simulink library "bcm"  (R2021b)
settings: Solver=VariableStepAuto  StartTime=0.0  StopTime=10.0  RelTol=1e-3
undefined symbols (not defined in the file or in its folder): ENUM_ANTITHEFT_ALARM, ENUM_ANTITHEFT_ARM, ENUM_ANTITHEFT_DISARM, ENUM_ANTITHEFT_WAIT, ENUM_GEARPOSNTOCAN_P, ENUM_PDKEYRAWLULOCK_INUNLOCK, ENUM_PDKEYRAWPS_INPS, ENUM_POWERSTA_ON, ENUM_POWERSTA_READY, ENUM_POWERSTA_STANDBY, ENUM_PWRSTASW_ON, ENUM_PWRSTASW_READY, ENUM_VEHICLETYPE_D21, ENUM_VEHICLETYPE_D31F25, ENUM_VEHICLETYPE_D31HAWD, ENUM_VEHICLETYPE_D31HRWD, ENUM_VEHICLETYPE_D31L24, FALSE, KBCM_ACCSwcPrsTmr_s, KBCM_ALMBrightnessDark_enum, KBCM_AmbBlue_enum, KBCM_AmbBreathT_ms, KBCM_AmbGreen_enum, KBCM_AmbMidPple_enum, KBCM_AmbRed_enum, KBCM_AmbTempCtrlEN_flg, KBCM_AmbTempT_s, KBCM_AmbWelModeENWait_s, KBCM_Antitheft_enum_ovrdflg, KBCM_Antitheft_enum_ovrdval, KBCM_APMDoorCtrlSta_flg_ovrdflg, KBCM_APMDoorCtrlSta_flg_ovrdval, KBCM_CmdKeepT_s, KBCM_CSWLightRstDebT_s, KBCM_CSWTurnLPRstT_s, KBCM_DelayTSW_flg, KBCM_DiagDRLOFF_flg, KBCM_DiagFLTC_mA, KBCM_DiagFMHT_s, KBCM_DiagFRTC_mA, KBCM_DiagRLTC_mA, KBCM_DiagRRTC_mA, KBCM_DrAPMRetryTimes_cnt, KBCM_DrOpenWdwOT_s, KBCM_DrOpenWdwReady_s, KBCM_ESSOffT_ms, KBCM_ESSOnT_ms, KBCM_FDCDKCReDetectT_K, KBCM_FDCDKCUSSFilterT_K, KBCM_HandleLampKeepT_s, KBCM_IVIRstHoldT_ms, KBCM_IVIRstTriggerT_ms, KBCM_ONDelayT_ms, KBCM_RAPSAbnFlashOFFT_ms, KBCM_RAPSAbnFlashONT_ms, KBCM_ReDetectT_K, KBCM_RightHandDriveEN_flg, KBCM_RLSLowSpdFilterT_s, KBCM_RmLampKeep_min, KBCM_RmLpKeyInT_s ... (+37)
libraries: simulink x447, $bdroot x11, hcu_lib x2
(part 7 of 13)

== system bcm/BCM/BCM/Personal_Setting/PTG ==
  note: Remove_After_Account_Switch_Function_Applied
  UserNow : Inport
  Loadbar : Inport  Port=2
  VINP_IVIPTGOpenHeight_enum : Inport  Port=3
  VINP_FlashPTGOpenHeight12_enum : Inport  Port=4
  VINP_FlashPTGOpenHeight34_enum : Inport  Port=5
  VINP_FlashPTGOpenHeight57_enum : Inport  Port=6
  VINP_PTGIsSetHeight_flg : Inport  Port=7
  VINP_BPPTGIsSetHeightSta_flg : Inport  Port=8
  VINP_PTGLeftHallPosn_cnt : Inport  Port=9
  VINP_FlashPTGUserHeight1_cnt : Inport  Port=10
  VINP_FlashPTGUserHeight2_cnt : Inport  Port=11
  VINP_FlashPTGUserHeight3_cnt : Inport  Port=12
  VINP_FlashPTGUserHeight4_cnt : Inport  Port=13
  VINP_FlashPTGUserHeight5_cnt : Inport  Port=14
  VINP_FlashPTGUserHeight7_cnt : Inport  Port=15
  VINP_CANMsgValidIVI2_flg : Inport  Port=16
  VINP_CANMsgValidBodyZonePS1_flg : Inport  Port=17
  VINP_LeftHallPos_cnt : Inport  Port=18
  VINP_VehicleType_enum : Inport  Port=19
  Compare To Constant : simulink/Logic and Bit Operations/Compare To Constant  relop=<=  const=0  OutDataTypeStr=boolean
  Compare To Constant1 : simulink/Logic and Bit Operations/Compare To Constant  relop=<=  const=0  OutDataTypeStr=boolean
  Compare To Constant2 : simulink/Logic and Bit Operations/Compare To Constant  relop=>=  const=1023  OutDataTypeStr=boolean
  Constant : Constant  Value=1023
  Constant10 : Constant  Value=ENUM_VEHICLETYPE_D21
  Constant11 : Constant  Value=680
  Constant12 : Constant  Value=520
  Constant6 : Constant  Value=5
  Constant7 : Constant  Value=ZERO_INT
  Constant9 : Constant  Value=1023
  Data Type Conversion{1,7..10,14} (6 alike) : DataTypeConversion  OutDataTypeStr=uint16
  Data Type Conversion6 : DataTypeConversion  OutDataTypeStr=uint8
  Equal : RelationalOperator  Operator===  OutDataTypeStr=boolean  RndMeth=Simplest
  OR : Logic  Operator=OR  AllPortsSameDT=off  OutDataTypeStr=boolean
  Switch{,1,3..4} (4 alike) : Switch  Criteria=u2 ~= 0
  Switch2 : Switch  Criteria=u2 > Threshold
  VALUE_TYPE_FlasherSignal : Subsystem
  VALUE_TYPE_PTGUserSetMaxHeight : Subsystem
  VBCM_PTGOpenHeightSta_enum : Outport
  VBCM_UserHeightSet_cnt : Outport  Port=2
  VBCM_PTGUserHeight1_cnt : Outport  Port=3
  VBCM_PTGUserHeight2_cnt : Outport  Port=4
  VBCM_PTGUserHeight3_cnt : Outport  Port=5
  VBCM_PTGUserHeight4_cnt : Outport  Port=6
  VBCM_PTGUserHeight5_cnt : Outport  Port=7
  VBCM_PTGUserHeight7_cnt : Outport  Port=8
  VBCM_PTGOpenHeight12_enum : Outport  Port=9
  VBCM_PTGOpenHeight34_enum : Outport  Port=10
  VBCM_PTGOpenHeight57_enum : Outport  Port=11
  wires:
  Data Type Conversion1/1 -> VALUE_TYPE_PTGUserSetMaxHeight/11(NoReqV)
  VINP_FlashPTGUserHeight7_cnt/1 -> VALUE_TYPE_PTGUserSetMaxHeight/10(EEP_Set7)
  VINP_FlashPTGUserHeight5_cnt/1 -> VALUE_TYPE_PTGUserSetMaxHeight/9(EEP_Set5)
  VINP_FlashPTGUserHeight4_cnt/1 -> VALUE_TYPE_PTGUserSetMaxHeight/8(EEP_Set4)
  VINP_FlashPTGUserHeight3_cnt/1 -> VALUE_TYPE_PTGUserSetMaxHeight/7(EEP_Set3)
  VINP_FlashPTGUserHeight2_cnt/1 -> VALUE_TYPE_PTGUserSetMaxHeight/6(EEP_Set2)
  VALUE_TYPE_PTGUserSetMaxHeight/7(Set7) -> VBCM_PTGUserHeight7_cnt/1
  VALUE_TYPE_PTGUserSetMaxHeight/6(Set5) -> VBCM_PTGUserHeight5_cnt/1
  VALUE_TYPE_PTGUserSetMaxHeight/5(Set4) -> VBCM_PTGUserHeight4_cnt/1
  VALUE_TYPE_PTGUserSetMaxHeight/4(Set3) -> VBCM_PTGUserHeight3_cnt/1
  VALUE_TYPE_PTGUserSetMaxHeight/3(Set2) -> VBCM_PTGUserHeight2_cnt/1
  VALUE_TYPE_PTGUserSetMaxHeight/2(Set1) -> VBCM_PTGUserHeight1_cnt/1
  VALUE_TYPE_PTGUserSetMaxHeight/1(Setting) -> VBCM_UserHeightSet_cnt/1
  Constant/1 -> Data Type Conversion1/1
  [Loadbar] -> VALUE_TYPE_PTGUserSetMaxHeight/2(Loadbar)
  [UserNow] -> VALUE_TYPE_PTGUserSetMaxHeight/1(UserNow)
  Loadbar/1 -> [Loadbar]
  UserNow/1 -> [UserNow]
  [UserNow] -> VALUE_TYPE_FlasherSignal/1(UserNow)
  [Loadbar] -> VALUE_TYPE_FlasherSignal/2(Loadbar)
  VINP_IVIPTGOpenHeight_enum/1 -> VALUE_TYPE_FlasherSignal/3(iviCMD)
  VALUE_TYPE_FlasherSignal/1(Setting) -> VBCM_PTGOpenHeightSta_enum/1
  Constant6/1 -> Data Type Conversion6/1
  Data Type Conversion6/1 -> VALUE_TYPE_FlasherSignal/8(NoReqV)
  VALUE_TYPE_FlasherSignal/2(Set12) -> VBCM_PTGOpenHeight12_enum/1
  VALUE_TYPE_FlasherSignal/3(Set34) -> VBCM_PTGOpenHeight34_enum/1
  VALUE_TYPE_FlasherSignal/4(Set57) -> VBCM_PTGOpenHeight57_enum/1
  VINP_FlashPTGOpenHeight34_enum/1 -> VALUE_TYPE_FlasherSignal/5(EEP_Set34)
  VINP_FlashPTGOpenHeight57_enum/1 -> VALUE_TYPE_FlasherSignal/6(EEP_Set57)
  VINP_CANMsgValidIVI2_flg/1 -> VALUE_TYPE_FlasherSignal/7(VINP_CANMsgValidIVI2_flg)
  VINP_FlashPTGOpenHeight12_enum/1 -> VALUE_TYPE_FlasherSignal/4(EEP_Set12)
  Switch4/1 -> [VBCM_PTGIsSetHeight_flg]
  Switch/1 -> [VBCM_PTGLeftHallPosn_cnt]  "VBCM_PTGLeftHallPosn_cnt"
  VINP_PTGLeftHallPosn_cnt/1 -> Data Type Conversion14/1
  VINP_PTGIsSetHeight_flg/1 -> Switch4/3
  [VINP_CANMsgValidBodyZonePS1_flg] -> Switch/2
  [VINP_CANMsgValidBodyZonePS1_flg] -> Switch4/2
  Switch3/1 -> [VBCM_FlashPTGUserHeight1_cnt]
  [VBCM_PTGDefMaxOpenHeight_cnt] -> Switch3/1
  Compare To Constant1/1 -> Switch3/2
  Data Type Conversion14/1 -> Switch/1
  VINP_BPPTGIsSetHeightSta_flg/1 -> Switch4/1
  [VBCM_FlashPTGUserHeight1_cnt] -> VALUE_TYPE_PTGUserSetMaxHeight/5(EEP_Set1)
  VINP_FlashPTGUserHeight1_cnt/1 -> Switch3/3, Compare To Constant1/1
  [VBCM_PTGLeftHallPosn_cnt] -> VALUE_TYPE_PTGUserSetMaxHeight/4(VINP_PTGLeftHallPosn_cnt)
  [VBCM_PTGIsSetHeight_flg] -> VALUE_TYPE_PTGUserSetMaxHeight/3(VINP_PTGIsSetHeightSta_flg)
  VINP_CANMsgValidBodyZonePS1_flg/1 -> [VINP_CANMsgValidBodyZonePS1_flg]
  Switch1/1 -> Switch/3  "VBCM_PTGLeftHallPosn_cnt"
  OR/1 -> Switch1/2
  Compare To Constant/1 -> OR/1
  VINP_LeftHallPos_cnt/1 -> Data Type Conversion10/1, Compare To Constant2/1, Compare To Constant/1
  Compare To Constant2/1 -> OR/2
  Data Type Conversion9/1 -> Switch1/1
  Data Type Conversion10/1 -> Switch1/3
  Constant9/1 -> Data Type Conversion9/1
  Constant7/1 -> VALUE_TYPE_FlasherSignal/9(Default)
  VINP_VehicleType_enum/1 -> [VINP_VehicleType_enum]
  [VINP_VehicleType_enum] -> Equal/1
  Constant10/1 -> Equal/2
  Equal/1 -> Switch2/2
  Data Type Conversion8/1 -> Switch2/3
  Data Type Conversion7/1 -> Switch2/1
  Constant11/1 -> Data Type Conversion7/1
  Constant12/1 -> Data Type Conversion8/1
  Switch2/1 -> [VBCM_PTGDefMaxOpenHeight_cnt]
  [VBCM_PTGDefMaxOpenHeight_cnt] -> VALUE_TYPE_PTGUserSetMaxHeight/12(Default)

== system bcm/BCM/BCM/Personal_Setting/RoomLamp ==
  UserNow : Inport
  Loadbar : Inport  Port=2
  VINP_RoomLampMode_flg : Inport  Port=3
  VINP_FlashRmLpModeEN_enum : Inport  Port=4
  VINP_SWC2RCustomizeSta_flg : Inport  Port=5
  VINP_IVISWCRUndefinedSta_enum : Inport  Port=6
  HMI_AutoInterLight_Cmd : Inport  Port=7
  AND : Logic  AllPortsSameDT=off  OutDataTypeStr=boolean
  AND1 : Logic  Operator=OR  Inputs=3  AllPortsSameDT=off  OutDataTypeStr=boolean
  Compare To Constant : simulink/Logic and Bit Operations/Compare To Constant  relop===  const=2  OutDataTypeStr=boolean
  Constant : Constant  OutDataTypeStr=boolean
  Detect Increase : simulink/Logic and Bit Operations/Detect Increase  vinit=0.0  OutDataTypeStr=boolean
  Detect Increase1 : simulink/Logic and Bit Operations/Detect Increase  vinit=0.0  OutDataTypeStr=boolean
  Detect Increase2 : simulink/Logic and Bit Operations/Detect Increase  vinit=0.0  OutDataTypeStr=boolean
  TOGGLE_TYPE_RoomLampMode : Subsystem
  FDC_BCM_RmLpModeENFun_Sta : Outport
  VBCM_RmLpModeENMem_enum : Outport  Port=2
  wires:
  TOGGLE_TYPE_RoomLampMode/1(Setting) -> FDC_BCM_RmLpModeENFun_Sta/1
  TOGGLE_TYPE_RoomLampMode/2(Set) -> VBCM_RmLpModeENMem_enum/1
  UserNow/1 -> [UserNow]
  Loadbar/1 -> [Loadbar]
  [UserNow] -> TOGGLE_TYPE_RoomLampMode/1(UserNow)
  [Loadbar] -> TOGGLE_TYPE_RoomLampMode/2(Loadbar)
  VINP_FlashRmLpModeEN_enum/1 -> TOGGLE_TYPE_RoomLampMode/4(EEP_Set)
  Constant/1 -> TOGGLE_TYPE_RoomLampMode/5(Default)
  VINP_IVISWCRUndefinedSta_enum/1 -> Compare To Constant/1
  VINP_SWC2RCustomizeSta_flg/1 -> Detect Increase/1
  HMI_AutoInterLight_Cmd/1 -> Detect Increase1/1
  Detect Increase/1 -> AND/1
  Compare To Constant/1 -> AND/2
  AND1/1 -> TOGGLE_TYPE_RoomLampMode/3(iviCMD)
  AND/1 -> AND1/2
  Detect Increase1/1 -> AND1/3
  VINP_RoomLampMode_flg/1 -> Detect Increase2/1
  Detect Increase2/1 -> AND1/1

== system bcm/BCM/BCM/Personal_Setting/SPTG ==
  UserNow : Inport
  Loadbar : Inport  Port=2
  VINP_IVIPTGUSStaSW_flg : Inport  Port=3
  VINP_FlashSPTGENFun_enum : Inport  Port=4
  Constant1 : Constant  OutDataTypeStr=boolean
  TOGGLE_TYPE_AmbFunEN : Subsystem
  FDC_SPTG_SPTGENFun_Sta : Outport
  VBCM_SPTGENFunMem_enum : Outport  Port=2
  wires:
  UserNow/1 -> TOGGLE_TYPE_AmbFunEN/1(UserNow)
  Loadbar/1 -> TOGGLE_TYPE_AmbFunEN/2(Loadbar)
  VINP_IVIPTGUSStaSW_flg/1 -> TOGGLE_TYPE_AmbFunEN/3(iviCMD)
  VINP_FlashSPTGENFun_enum/1 -> TOGGLE_TYPE_AmbFunEN/4(EEP_Set)
  Constant1/1 -> TOGGLE_TYPE_AmbFunEN/5(Default)
  TOGGLE_TYPE_AmbFunEN/1(Setting) -> FDC_SPTG_SPTGENFun_Sta/1
  TOGGLE_TYPE_AmbFunEN/2(Set) -> VBCM_SPTGENFunMem_enum/1

== system bcm/BCM/BCM/Personal_Setting/System_Loadbar ==
  Add : Sum
  Compare To Constant : simulink/Logic and Bit Operations/Compare To Constant  relop=>  const=2  OutDataTypeStr=boolean
  Constant6 : Constant  Value=0  OutDataTypeStr=uint8
  Constant7 : Constant  OutDataTypeStr=uint8
  Switch7 : Switch  Criteria=u2 > Threshold
  Unit Delay : UnitDelay  SampleTime=-1  HasFrameUpgradeWarning=on
  Unit Delay6 : UnitDelay  SampleTime=-1  HasFrameUpgradeWarning=on
  Loadbar : Outport
  wires:
  Constant7/1 -> Switch7/3
  Unit Delay6/1 -> Add/1
  Switch7/1 -> Add/2
  Unit Delay/1 -> Switch7/2
  Compare To Constant/1 -> Unit Delay/1, Loadbar/1
  Add/1 -> Unit Delay6/1, Compare To Constant/1
  Constant6/1 -> Switch7/1

== system bcm/BCM/BCM/Personal_Setting/Window ==
  UserNow : Inport
  Loadbar : Inport  Port=2
  UpdateReq : Inport  Port=3
  VINP_IVICLWinLockDrSW_flg : Inport  Port=4
  VINP_FlashCLWinLockDrSta_enum : Inport  Port=5
  Constant : Constant  Value=TRUE
  TOGGLE_TYPE_CLWinOWhenLock : $bdroot/BCM/BCM/Personal_Setting/Autolock/TOGGLE_TYPE_AutoLock  SystemSampleTime=-1  VariantActivationTime=update diagram  Latency=0  AutoFrameSizeCalculation=off
  VBCM_CLWinLockDrSta_flg : Outport
  VBCM_CLWinLockDrStaMem_enum : Outport  Port=2
  wires:
  Constant/1 -> TOGGLE_TYPE_CLWinOWhenLock/6
  UserNow/1 -> TOGGLE_TYPE_CLWinOWhenLock/1
  Loadbar/1 -> TOGGLE_TYPE_CLWinOWhenLock/2
  UpdateReq/1 -> TOGGLE_TYPE_CLWinOWhenLock/3
  VINP_IVICLWinLockDrSW_flg/1 -> TOGGLE_TYPE_CLWinOWhenLock/4
  VINP_FlashCLWinLockDrSta_enum/1 -> TOGGLE_TYPE_CLWinOWhenLock/5
  TOGGLE_TYPE_CLWinOWhenLock/1 -> VBCM_CLWinLockDrSta_flg/1  "VBCM_CLWinLockDrSta_flg"
  TOGGLE_TYPE_CLWinOWhenLock/2 -> VBCM_CLWinLockDrStaMem_enum/1  "VBCM_CLWinLockDrStaMem_enum"

== system bcm/BCM/BCM/WasherWiper/RLS_Command_Cut_Filter ==
  VINP_RLSRainSnrWiperCmd_enum : Inport
  task_time_s : Inport  Port=2
  VINP_DiagWipRLSCmdCutEN_flg : Inport  Port=3
  VINP_DiagRLSCmdCutTime_s : Inport  Port=4
  Add : Sum
  Add1 : Sum
  Constant : Constant  Value=2
  Constant1 : Constant  Value=3
  Constant10 : Constant  Value=ONE_INT16
  Constant2 : Constant  Value=ZERO_INT16
  Constant3 : Constant  Value=ONE_INT16
  Constant4 : Constant  Value=3
  Constant5 : Constant  Value=3
  Constant8 : Constant  Value=KBCM_RLSLowSpdFilterT_s
  Constant9 : Constant  Value=ZERO_INT16
  Data Type Conversion : DataTypeConversion  OutDataTypeStr=single
  Data Type Conversion{1..2,5..6} (4 alike) : DataTypeConversion  OutDataTypeStr=uint8
  Data Type Conversion9 : DataTypeConversion  OutDataTypeStr=uint16
  Divide : Product  Inputs=*/
  Divide1 : Product  Inputs=*/
  Equal : RelationalOperator  Operator===  OutDataTypeStr=boolean  RndMeth=Simplest
  Equal1 : RelationalOperator  Operator===  OutDataTypeStr=boolean  RndMeth=Simplest
  Less Than : RelationalOperator  Operator=>  OutDataTypeStr=boolean  RndMeth=Simplest
  OR : Logic  Operator=OR  AllPortsSameDT=off  OutDataTypeStr=boolean
  Relational Operator : RelationalOperator  Operator===  OutDataTypeStr=boolean  RndMeth=Simplest
  Relational Operator1 : RelationalOperator  Operator=>  OutDataTypeStr=boolean  RndMeth=Simplest
  Saturation : Saturate  UpperLimit=1000  LowerLimit=0
  Saturation1 : Saturate  UpperLimit=65500  LowerLimit=0
  Switch : Switch  Criteria=u2 ~= 0
  Switch{1..6} (6 alike) : Switch  Criteria=u2 > Threshold
  Unit Delay{,1..3} (4 alike) : UnitDelay  SampleTime=-1  HasFrameUpgradeWarning=on
  RLS_WiperCmd : Outport
  wires:
  Data Type Conversion5/1 -> Switch3/1
  Unit Delay2/1 -> Switch4/1
  Constant5/1 -> Data Type Conversion5/1
  Switch2/1 -> Saturation/1
  Add/1 -> Switch2/1
  VINP_RLSRainSnrWiperCmd_enum/1 -> [VINP_RLSRainSnrWiperCmd_enum]
  Switch4/1 -> Switch3/3, Unit Delay2/1
  [VINP_RLSRainSnrWiperCmd_enum] -> Switch4/3
  Relational Operator1/1 -> Switch3/2
  Unit Delay1/1 -> Add/1
  Data Type Conversion2/1 -> Relational Operator/2
  [VINP_RLSRainSnrWiperCmd_enum] -> Relational Operator/1
  Constant1/1 -> Data Type Conversion2/1
  Relational Operator/1 -> Switch4/2, Switch2/2
  Saturation/1 -> Relational Operator1/1, Unit Delay1/1
  Divide/1 -> Relational Operator1/2
  VINP_DiagRLSCmdCutTime_s/1 -> Data Type Conversion/1
  VINP_DiagWipRLSCmdCutEN_flg/1 -> Switch/2
  Switch3/1 -> Switch/1
  [VINP_RLSRainSnrWiperCmd_enum] -> Switch/3
  Data Type Conversion/1 -> Divide/1
  [VINP_RLSRainSnrWiperCmd_enum] -> Equal/1
  Constant/1 -> Data Type Conversion1/1
  Data Type Conversion1/1 -> Equal/2
  Data Type Conversion6/1 -> Equal1/2
  Constant4/1 -> Data Type Conversion6/1
  [VINP_RLSRainSnrWiperCmd_enum] -> Equal1/1
  Equal/1 -> OR/1
  Equal1/1 -> OR/2
  OR/1 -> Switch5/2, Switch1/2
  Add1/1 -> Switch1/1
  Unit Delay/1 -> Add1/1
  Switch1/1 -> Saturation1/1
  Saturation1/1 -> Less Than/1, Unit Delay/1
  Switch5/1 -> Unit Delay3/1, Switch6/3
  Unit Delay3/1 -> Switch5/1
  Data Type Conversion9/1 -> Less Than/2
  Less Than/1 -> Switch6/2
  Switch6/1 -> RLS_WiperCmd/1
  Switch/1 -> Switch5/3, Switch6/1
  task_time_s/1 -> [task_time_s]
  [task_time_s] -> Divide/2
  Constant8/1 -> Divide1/1
  [task_time_s] -> Divide1/2
  Divide1/1 -> Data Type Conversion9/1
  Constant10/1 -> Add/2
  Constant9/1 -> Switch2/3
  Constant2/1 -> Switch1/3
  Constant3/1 -> Add1/2

== system bcm/BCM/BCM/Window_Control_Sig_Combine/Driver_Window ==
  note: 0:NoReq
      | 1:BCM
      | 2.IVI
      | 3:DKC
      | 4:CONN
  note: 0:NoReq
      | 1:BCM
      | 2.IVI
      | 3:DKC
      | 4:CONN
  DKCWINCMD : Inport
  IVIWINCMD : Inport  Port=2
  CONNWINCMD : Inport  Port=3
  BCMWINCMD : Inport  Port=4
  Add{,1..3} (4 alike) : Sum  Inputs=-+
  Compare To Constant{,1..3} (4 alike) : simulink/Logic and Bit Operations/Compare To Constant  relop=>  const=0  OutDataTypeStr=boolean
  Constant{,1..3} (4 alike) : Constant  Value=100
  Constant10 : Constant  Value=127
  Constant{11,13,15,17} (4 alike) : Constant  Value=10
  Constant{8,12,14,16,18} (5 alike) : Constant
  Constant4 : Constant  Value=0
  Constant5 : Constant  Value=4
  Constant6 : Constant  Value=2
  Constant7 : Constant  Value=3
  Constant9 : Constant  Value=127
  Data Type Conversion{,1..6} (7 alike) : DataTypeConversion  OutDataTypeStr=uint8
  Data Type Conversion{7..14} (8 alike) : DataTypeConversion  OutDataTypeStr=int8
  Detect Decrease{1..4} (4 alike) : simulink/Logic and Bit Operations/Detect Decrease  vinit=0.0  OutDataTypeStr=boolean
  Multiport Switch : MultiPortSwitch  DataPortOrder=Zero-based contiguous  Inputs=6  DiagnosticForDefault=None  zeroidx=on
  Relational Operator{,1..3} (4 alike) : RelationalOperator  Operator=>  OutDataTypeStr=boolean  RndMeth=Simplest
  Saturation{,1..3} (4 alike) : Saturate  UpperLimit=10  LowerLimit=0
  Switch{,1..7} (8 alike) : Switch  Criteria=u2 > Threshold
  Unit Delay{,1..3} (4 alike) : UnitDelay  SampleTime=-1  HasFrameUpgradeWarning=on
  WINCMD : Outport
  WINReqAP : Outport  Port=2
  wires:
  Constant7/1 -> Data Type Conversion3/1
  CONNWINCMD/1 -> [CONNWINCMD]
  [CONNWINCMD] -> Relational Operator2/1
  Constant5/1 -> Data Type Conversion1/1
  [WINReqAP] -> Multiport Switch/1
  [BCMReq] -> Switch3/2
  Constant10/1 -> Data Type Conversion6/1
  [DKCReq] -> Switch1/2
  Constant9/1 -> Data Type Conversion5/1
  [CONNReq] -> Switch/2
  [DKCWINCMD] -> Multiport Switch/5
  Constant8/1 -> Data Type Conversion4/1
  Data Type Conversion/1 -> Switch/3
  [BCMWINCMD] -> Multiport Switch/3
  Multiport Switch/1 -> WINCMD/1
  Data Type Conversion3/1 -> Switch1/1
  Data Type Conversion1/1 -> Switch/1
  Constant2/1 -> Relational Operator2/2
  Constant4/1 -> Data Type Conversion/1
  Constant3/1 -> Relational Operator3/2
  Data Type Conversion5/1 -> Multiport Switch/2
  DKCWINCMD/1 -> [DKCWINCMD]
  BCMWINCMD/1 -> [BCMWINCMD]
  IVIWINCMD/1 -> [IVIWINCMD]
  Constant/1 -> Relational Operator/2
  [DKCWINCMD] -> Relational Operator/1
  [IVIWINCMD] -> Multiport Switch/4
  [CONNWINCMD] -> Multiport Switch/6
  Constant1/1 -> Relational Operator1/2
  [BCMWINCMD] -> Relational Operator3/1
  Data Type Conversion4/1 -> Switch3/1
  Switch1/1 -> Switch2/3
  Switch/1 -> Switch1/3
  [IVIWINCMD] -> Relational Operator1/1
  Switch3/1 -> [WINReqAP]
  Switch2/1 -> Switch3/3
  Constant6/1 -> Data Type Conversion2/1
  Data Type Conversion2/1 -> Switch2/1
  [IVIReq] -> Switch2/2
  [WINReqAP] -> WINReqAP/1
  Data Type Conversion6/1 -> Multiport Switch/7
  Relational Operator/1 -> Detect Decrease4/1
  Saturation/1 -> Compare To Constant/1, Unit Delay/1
  Constant11/1 -> Data Type Conversion7/1
  Detect Decrease4/1 -> Switch4/2
  Unit Delay/1 -> Add/2
  Add/1 -> Switch4/3
  Data Type Conversion7/1 -> Switch4/1
  Data Type Conversion8/1 -> Add/1
  Constant12/1 -> Data Type Conversion8/1
  Switch4/1 -> Saturation/1
  Compare To Constant/1 -> [DKCReq]
  Compare To Constant1/1 -> [IVIReq]
  Switch5/1 -> Saturation1/1
  Constant14/1 -> Data Type Conversion10/1
  Data Type Conversion10/1 -> Add1/1
  Data Type Conversion9/1 -> Switch5/1
  Add1/1 -> Switch5/3
  Unit Delay1/1 -> Add1/2
  Detect Decrease1/1 -> Switch5/2
  Constant13/1 -> Data Type Conversion9/1
  Saturation1/1 -> Unit Delay1/1, Compare To Constant1/1
  Relational Operator1/1 -> Detect Decrease1/1
  Saturation2/1 -> Compare To Constant2/1, Unit Delay2/1
  Constant15/1 -> Data Type Conversion12/1
  Detect Decrease2/1 -> Switch6/2
  Unit Delay2/1 -> Add2/2
  Add2/1 -> Switch6/3
  Data Type Conversion12/1 -> Switch6/1
  Data Type Conversion11/1 -> Add2/1
  Constant16/1 -> Data Type Conversion11/1
  Switch6/1 -> Saturation2/1
  Compare To Constant2/1 -> [CONNReq]
  Relational Operator2/1 -> Detect Decrease2/1
  Compare To Constant3/1 -> [BCMReq]
  Switch7/1 -> Saturation3/1
  Constant18/1 -> Data Type Conversion13/1
  Data Type Conversion13/1 -> Add3/1
  Data Type Conversion14/1 -> Switch7/1
  Add3/1 -> Switch7/3
  Unit Delay3/1 -> Add3/2
  Detect Decrease3/1 -> Switch7/2
  Constant17/1 -> Data Type Conversion14/1
  Saturation3/1 -> Unit Delay3/1, Compare To Constant3/1
  Relational Operator3/1 -> Detect Decrease3/1

== system bcm/BCM/BCM/Window_Control_Sig_Combine/Passenger_Window ==
  note: 0:NoReq
      | 1:BCM
      | 2.IVI
      | 3:DKC
      | 4:CONN
  note: 0:NoReq
      | 1:BCM
      | 2.IVI
      | 3:DKC
      | 4:CONN
  DKCWINCMD : Inport
  IVIWINCMD : Inport  Port=2
  CONNWINCMD : Inport  Port=3
  BCMWINCMD : Inport  Port=4
  Add{,1..3} (4 alike) : Sum  Inputs=-+
  Compare To Constant{,1..3} (4 alike) : simulink/Logic and Bit Operations/Compare To Constant  relop=>  const=0  OutDataTypeStr=boolean
  Constant{,1..3} (4 alike) : Constant  Value=100
  Constant10 : Constant  Value=127
  Constant{11,13,15,17} (4 alike) : Constant  Value=10
  Constant{8,12,14,16,18} (5 alike) : Constant
  Constant4 : Constant  Value=0
  Constant5 : Constant  Value=4
  Constant6 : Constant  Value=2
  Constant7 : Constant  Value=3
  Constant9 : Constant  Value=127
  Data Type Conversion{,1..6} (7 alike) : DataTypeConversion  OutDataTypeStr=uint8
  Data Type Conversion{7..14} (8 alike) : DataTypeConversion  OutDataTypeStr=int8
  Detect Decrease{1..4} (4 alike) : simulink/Logic and Bit Operations/Detect Decrease  vinit=0.0  OutDataTypeStr=boolean
  Multiport Switch : MultiPortSwitch  DataPortOrder=Zero-based contiguous  Inputs=6  DiagnosticForDefault=None  zeroidx=on
  Relational Operator{,1..3} (4 alike) : RelationalOperator  Operator=>  OutDataTypeStr=boolean  RndMeth=Simplest
  Saturation{,1..3} (4 alike) : Saturate  UpperLimit=10  LowerLimit=0
  Switch{,1..7} (8 alike) : Switch  Criteria=u2 > Threshold
  Unit Delay{,1..3} (4 alike) : UnitDelay  SampleTime=-1  HasFrameUpgradeWarning=on
  WINCMD : Outport
  WINReqAP : Outport  Port=2
  wires:
  Relational Operator3/1 -> Detect Decrease3/1
  Saturation3/1 -> Compare To Constant3/1, Unit Delay3/1
  Constant17/1 -> Data Type Conversion14/1
  Detect Decrease3/1 -> Switch7/2
  Unit Delay3/1 -> Add3/2
  Add3/1 -> Switch7/3
  Data Type Conversion14/1 -> Switch7/1
  Data Type Conversion13/1 -> Add3/1
  Constant18/1 -> Data Type Conversion13/1
  Switch7/1 -> Saturation3/1
  Compare To Constant3/1 -> [BCMReq]
  Relational Operator2/1 -> Detect Decrease2/1
  Compare To Constant2/1 -> [CONNReq]
  Switch6/1 -> Saturation2/1
  Constant16/1 -> Data Type Conversion11/1
  Data Type Conversion11/1 -> Add2/1
  Data Type Conversion12/1 -> Switch6/1
  Add2/1 -> Switch6/3
  Unit Delay2/1 -> Add2/2
  Detect Decrease2/1 -> Switch6/2
  Constant15/1 -> Data Type Conversion12/1
  Saturation2/1 -> Unit Delay2/1, Compare To Constant2/1
  Relational Operator1/1 -> Detect Decrease1/1
  Saturation1/1 -> Compare To Constant1/1, Unit Delay1/1
  Constant13/1 -> Data Type Conversion9/1
  Detect Decrease1/1 -> Switch5/2
  Unit Delay1/1 -> Add1/2
  Add1/1 -> Switch5/3
  Data Type Conversion9/1 -> Switch5/1
  Data Type Conversion10/1 -> Add1/1
  Constant14/1 -> Data Type Conversion10/1
  Switch5/1 -> Saturation1/1
  Compare To Constant1/1 -> [IVIReq]
  Compare To Constant/1 -> [DKCReq]
  Switch4/1 -> Saturation/1
  Constant12/1 -> Data Type Conversion8/1
  Data Type Conversion8/1 -> Add/1
  Data Type Conversion7/1 -> Switch4/1
  Add/1 -> Switch4/3
  Unit Delay/1 -> Add/2
  Detect Decrease4/1 -> Switch4/2
  Constant11/1 -> Data Type Conversion7/1
  Saturation/1 -> Unit Delay/1, Compare To Constant/1
  Relational Operator/1 -> Detect Decrease4/1
  Data Type Conversion6/1 -> Multiport Switch/7
  [WINReqAP] -> WINReqAP/1
  [IVIReq] -> Switch2/2
  Data Type Conversion2/1 -> Switch2/1
  Constant6/1 -> Data Type Conversion2/1
  Switch2/1 -> Switch3/3
  Switch3/1 -> [WINReqAP]
  [IVIWINCMD] -> Relational Operator1/1
  Switch/1 -> Switch1/3
  Switch1/1 -> Switch2/3
  Data Type Conversion4/1 -> Switch3/1
  [BCMWINCMD] -> Relational Operator3/1
  Constant1/1 -> Relational Operator1/2
  [CONNWINCMD] -> Multiport Switch/6
  [IVIWINCMD] -> Multiport Switch/4
  [DKCWINCMD] -> Relational Operator/1
  Constant/1 -> Relational Operator/2
  IVIWINCMD/1 -> [IVIWINCMD]
  BCMWINCMD/1 -> [BCMWINCMD]
  DKCWINCMD/1 -> [DKCWINCMD]
  Data Type Conversion5/1 -> Multiport Switch/2
  Constant3/1 -> Relational Operator3/2
  Constant4/1 -> Data Type Conversion/1
  Constant2/1 -> Relational Operator2/2
  Data Type Conversion1/1 -> Switch/1
  Data Type Conversion3/1 -> Switch1/1
  Multiport Switch/1 -> WINCMD/1
  [BCMWINCMD] -> Multiport Switch/3
  Data Type Conversion/1 -> Switch/3
  Constant8/1 -> Data Type Conversion4/1
  [DKCWINCMD] -> Multiport Switch/5
  [CONNReq] -> Switch/2
  Constant9/1 -> Data Type Conversion5/1
  [DKCReq] -> Switch1/2
  Constant10/1 -> Data Type Conversion6/1
  [BCMReq] -> Switch3/2
  [WINReqAP] -> Multiport Switch/1
  Constant5/1 -> Data Type Conversion1/1
  [CONNWINCMD] -> Relational Operator2/1
  CONNWINCMD/1 -> [CONNWINCMD]
  Constant7/1 -> Data Type Conversion3/1

== system bcm/BCM/BCM/Window_Control_Sig_Combine/RearLeft_Window ==
  note: 0:NoReq
      | 1:BCM
      | 2.IVI
      | 3:DKC
      | 4:CONN
  note: 0:NoReq
      | 1:BCM
      | 2.IVI
      | 3:DKC
      | 4:CONN
  DKCWINCMD : Inport
  IVIWINCMD : Inport  Port=2
  CONNWINCMD : Inport  Port=3
  BCMWINCMD : Inport  Port=4
  Add{,1..3} (4 alike) : Sum  Inputs=-+
  Compare To Constant{,1..3} (4 alike) : simulink/Logic and Bit Operations/Compare To Constant  relop=>  const=0  OutDataTypeStr=boolean
  Constant{,1..3} (4 alike) : Constant  Value=100
  Constant10 : Constant  Value=127
  Constant{11,13,15,17} (4 alike) : Constant  Value=10
  Constant{8,12,14,16,18} (5 alike) : Constant
  Constant4 : Constant  Value=0
  Constant5 : Constant  Value=4
  Constant6 : Constant  Value=2
  Constant7 : Constant  Value=3
  Constant9 : Constant  Value=127
  Data Type Conversion{,1..6} (7 alike) : DataTypeConversion  OutDataTypeStr=uint8
  Data Type Conversion{7..14} (8 alike) : DataTypeConversion  OutDataTypeStr=int8
  Detect Decrease{1..4} (4 alike) : simulink/Logic and Bit Operations/Detect Decrease  vinit=0.0  OutDataTypeStr=boolean
  Multiport Switch : MultiPortSwitch  DataPortOrder=Zero-based contiguous  Inputs=6  DiagnosticForDefault=None  zeroidx=on
  Relational Operator{,1..3} (4 alike) : RelationalOperator  Operator=>  OutDataTypeStr=boolean  RndMeth=Simplest
  Saturation{,1..3} (4 alike) : Saturate  UpperLimit=10  LowerLimit=0
  Switch{,1..7} (8 alike) : Switch  Criteria=u2 > Threshold
  Unit Delay{,1..3} (4 alike) : UnitDelay  SampleTime=-1  HasFrameUpgradeWarning=on
  WINCMD : Outport
  WINReqAP : Outport  Port=2
  wires:
  Relational Operator3/1 -> Detect Decrease3/1
  Saturation3/1 -> Compare To Constant3/1, Unit Delay3/1
  Constant17/1 -> Data Type Conversion14/1
  Detect Decrease3/1 -> Switch7/2
  Unit Delay3/1 -> Add3/2
  Add3/1 -> Switch7/3
  Data Type Conversion14/1 -> Switch7/1
  Data Type Conversion13/1 -> Add3/1
  Constant18/1 -> Data Type Conversion13/1
  Switch7/1 -> Saturation3/1
  Compare To Constant3/1 -> [BCMReq]
  Relational Operator2/1 -> Detect Decrease2/1
  Compare To Constant2/1 -> [CONNReq]
  Switch6/1 -> Saturation2/1
  Constant16/1 -> Data Type Conversion11/1
  Data Type Conversion11/1 -> Add2/1
  Data Type Conversion12/1 -> Switch6/1
  Add2/1 -> Switch6/3
  Unit Delay2/1 -> Add2/2
  Detect Decrease2/1 -> Switch6/2
  Constant15/1 -> Data Type Conversion12/1
  Saturation2/1 -> Unit Delay2/1, Compare To Constant2/1
  Relational Operator1/1 -> Detect Decrease1/1
  Saturation1/1 -> Compare To Constant1/1, Unit Delay1/1
  Constant13/1 -> Data Type Conversion9/1
  Detect Decrease1/1 -> Switch5/2
  Unit Delay1/1 -> Add1/2
  Add1/1 -> Switch5/3
  Data Type Conversion9/1 -> Switch5/1
  Data Type Conversion10/1 -> Add1/1
  Constant14/1 -> Data Type Conversion10/1
  Switch5/1 -> Saturation1/1
  Compare To Constant1/1 -> [IVIReq]
  Compare To Constant/1 -> [DKCReq]
  Switch4/1 -> Saturation/1
  Constant12/1 -> Data Type Conversion8/1
  Data Type Conversion8/1 -> Add/1
  Data Type Conversion7/1 -> Switch4/1
  Add/1 -> Switch4/3
  Unit Delay/1 -> Add/2
  Detect Decrease4/1 -> Switch4/2
  Constant11/1 -> Data Type Conversion7/1
  Saturation/1 -> Unit Delay/1, Compare To Constant/1
  Relational Operator/1 -> Detect Decrease4/1
  Data Type Conversion6/1 -> Multiport Switch/7
  [WINReqAP] -> WINReqAP/1
  [IVIReq] -> Switch2/2
  Data Type Conversion2/1 -> Switch2/1
  Constant6/1 -> Data Type Conversion2/1
  Switch2/1 -> Switch3/3
  Switch3/1 -> [WINReqAP]
  [IVIWINCMD] -> Relational Operator1/1
  Switch/1 -> Switch1/3
  Switch1/1 -> Switch2/3
  Data Type Conversion4/1 -> Switch3/1
  [BCMWINCMD] -> Relational Operator3/1
  Constant1/1 -> Relational Operator1/2
  [CONNWINCMD] -> Multiport Switch/6
  [IVIWINCMD] -> Multiport Switch/4
  [DKCWINCMD] -> Relational Operator/1
  Constant/1 -> Relational Operator/2
  IVIWINCMD/1 -> [IVIWINCMD]
  BCMWINCMD/1 -> [BCMWINCMD]
  DKCWINCMD/1 -> [DKCWINCMD]
  Data Type Conversion5/1 -> Multiport Switch/2
  Constant3/1 -> Relational Operator3/2
  Constant4/1 -> Data Type Conversion/1
  Constant2/1 -> Relational Operator2/2
  Data Type Conversion1/1 -> Switch/1
  Data Type Conversion3/1 -> Switch1/1
  Multiport Switch/1 -> WINCMD/1
  [BCMWINCMD] -> Multiport Switch/3
  Data Type Conversion/1 -> Switch/3
  Constant8/1 -> Data Type Conversion4/1
  [DKCWINCMD] -> Multiport Switch/5
  [CONNReq] -> Switch/2
  Constant9/1 -> Data Type Conversion5/1
  [DKCReq] -> Switch1/2
  Constant10/1 -> Data Type Conversion6/1
  [BCMReq] -> Switch3/2
  [WINReqAP] -> Multiport Switch/1
  Constant5/1 -> Data Type Conversion1/1
  [CONNWINCMD] -> Relational Operator2/1
  CONNWINCMD/1 -> [CONNWINCMD]
  Constant7/1 -> Data Type Conversion3/1

== system bcm/BCM/BCM/Window_Control_Sig_Combine/RearRight_Window ==
  note: 0:NoReq
      | 1:BCM
      | 2.IVI
      | 3:DKC
      | 4:CONN
  note: 0:NoReq
      | 1:BCM
      | 2.IVI
      | 3:DKC
      | 4:CONN
  DKCWINCMD : Inport
  IVIWINCMD : Inport  Port=2
  CONNWINCMD : Inport  Port=3
  BCMWINCMD : Inport  Port=4
  Add{,1..3} (4 alike) : Sum  Inputs=-+
  Compare To Constant{,1..3} (4 alike) : simulink/Logic and Bit Operations/Compare To Constant  relop=>  const=0  OutDataTypeStr=boolean
  Constant{,1..3} (4 alike) : Constant  Value=100
  Constant10 : Constant  Value=127
  Constant{11,13,15,17} (4 alike) : Constant  Value=10
  Constant{8,12,14,16,18} (5 alike) : Constant
  Constant4 : Constant  Value=0
  Constant5 : Constant  Value=4
  Constant6 : Constant  Value=2
  Constant7 : Constant  Value=3
  Constant9 : Constant  Value=127
  Data Type Conversion{,1..6} (7 alike) : DataTypeConversion  OutDataTypeStr=uint8
  Data Type Conversion{7..14} (8 alike) : DataTypeConversion  OutDataTypeStr=int8
  Detect Decrease{1..4} (4 alike) : simulink/Logic and Bit Operations/Detect Decrease  vinit=0.0  OutDataTypeStr=boolean
  Multiport Switch : MultiPortSwitch  DataPortOrder=Zero-based contiguous  Inputs=6  DiagnosticForDefault=None  zeroidx=on
  Relational Operator{,1..3} (4 alike) : RelationalOperator  Operator=>  OutDataTypeStr=boolean  RndMeth=Simplest
  Saturation{,1..3} (4 alike) : Saturate  UpperLimit=10  LowerLimit=0
  Switch{,1..7} (8 alike) : Switch  Criteria=u2 > Threshold
  Unit Delay{,1..3} (4 alike) : UnitDelay  SampleTime=-1  HasFrameUpgradeWarning=on
  WINCMD : Outport
  WINReqAP : Outport  Port=2
  wires:
  Constant7/1 -> Data Type Conversion3/1
  CONNWINCMD/1 -> [CONNWINCMD]
  [CONNWINCMD] -> Relational Operator2/1
  Constant5/1 -> Data Type Conversion1/1
  [WINReqAP] -> Multiport Switch/1
  [BCMReq] -> Switch3/2
  Constant10/1 -> Data Type Conversion6/1
  [DKCReq] -> Switch1/2
  Constant9/1 -> Data Type Conversion5/1
  [CONNReq] -> Switch/2
  [DKCWINCMD] -> Multiport Switch/5
  Constant8/1 -> Data Type Conversion4/1
  Data Type Conversion/1 -> Switch/3
  [BCMWINCMD] -> Multiport Switch/3
  Multiport Switch/1 -> WINCMD/1
  Data Type Conversion3/1 -> Switch1/1
  Data Type Conversion1/1 -> Switch/1
  Constant2/1 -> Relational Operator2/2
  Constant4/1 -> Data Type Conversion/1
  Constant3/1 -> Relational Operator3/2
  Data Type Conversion5/1 -> Multiport Switch/2
  DKCWINCMD/1 -> [DKCWINCMD]
  BCMWINCMD/1 -> [BCMWINCMD]
  IVIWINCMD/1 -> [IVIWINCMD]
  Constant/1 -> Relational Operator/2
  [DKCWINCMD] -> Relational Operator/1
  [IVIWINCMD] -> Multiport Switch/4
  [CONNWINCMD] -> Multiport Switch/6
  Constant1/1 -> Relational Operator1/2
  [BCMWINCMD] -> Relational Operator3/1
  Data Type Conversion4/1 -> Switch3/1
  Switch1/1 -> Switch2/3
  Switch/1 -> Switch1/3
  [IVIWINCMD] -> Relational Operator1/1
  Switch3/1 -> [WINReqAP]
  Switch2/1 -> Switch3/3
  Constant6/1 -> Data Type Conversion2/1
  Data Type Conversion2/1 -> Switch2/1
  [IVIReq] -> Switch2/2
  [WINReqAP] -> WINReqAP/1
  Data Type Conversion6/1 -> Multiport Switch/7
  Relational Operator/1 -> Detect Decrease4/1
  Saturation/1 -> Compare To Constant/1, Unit Delay/1
  Constant11/1 -> Data Type Conversion7/1
  Detect Decrease4/1 -> Switch4/2
  Unit Delay/1 -> Add/2
  Add/1 -> Switch4/3
  Data Type Conversion7/1 -> Switch4/1
  Data Type Conversion8/1 -> Add/1
  Constant12/1 -> Data Type Conversion8/1
  Switch4/1 -> Saturation/1
  Compare To Constant/1 -> [DKCReq]
  Compare To Constant1/1 -> [IVIReq]
  Switch5/1 -> Saturation1/1
  Constant14/1 -> Data Type Conversion10/1
  Data Type Conversion10/1 -> Add1/1
  Data Type Conversion9/1 -> Switch5/1
  Add1/1 -> Switch5/3
  Unit Delay1/1 -> Add1/2
  Detect Decrease1/1 -> Switch5/2
  Constant13/1 -> Data Type Conversion9/1
  Saturation1/1 -> Unit Delay1/1, Compare To Constant1/1
  Relational Operator1/1 -> Detect Decrease1/1
  Saturation2/1 -> Compare To Constant2/1, Unit Delay2/1
  Constant15/1 -> Data Type Conversion12/1
  Detect Decrease2/1 -> Switch6/2
  Unit Delay2/1 -> Add2/2
  Add2/1 -> Switch6/3
  Data Type Conversion12/1 -> Switch6/1
  Data Type Conversion11/1 -> Add2/1
  Constant16/1 -> Data Type Conversion11/1
  Switch6/1 -> Saturation2/1
  Compare To Constant2/1 -> [CONNReq]
  Relational Operator2/1 -> Detect Decrease2/1
  Compare To Constant3/1 -> [BCMReq]
  Switch7/1 -> Saturation3/1
  Constant18/1 -> Data Type Conversion13/1
  Data Type Conversion13/1 -> Add3/1
  Data Type Conversion14/1 -> Switch7/1
  Add3/1 -> Switch7/3
  Unit Delay3/1 -> Add3/2
  Detect Decrease3/1 -> Switch7/2
  Constant17/1 -> Data Type Conversion14/1
  Saturation3/1 -> Unit Delay3/1, Compare To Constant3/1
  Relational Operator3/1 -> Detect Decrease3/1

== system bcm/BCM/BCM/PTG/KeyDetected/CheckSignalAvailable ==
  VBCM_PASDRML_cm_IN : Inport
  VBCM_PASDRMR_cm_IN : Inport  Port=2
  KBCM_USSDis_cm_IN : Inport  Port=3
  AND : Logic  Inputs=3  AllPortsSameDT=off  OutDataTypeStr=boolean
  Constant : Constant  OutDataTypeStr=single
  Constant1 : Constant  OutDataTypeStr=single
  Constant2 : Constant  OutDataTypeStr=single
  Constant3 : Constant  Value=KBCM_SPTGLowerBound_cm
  Constant4 : Constant  Value=KBCM_SPTGLowerBoundOut_cm
  Constant5 : Constant  Value=KBCM_SPTGLowerBound_cm
  Constant6 : Constant  Value=KBCM_SPTGLowerBoundOut_cm
  Demux : Demux  Outputs=3
  Equal : RelationalOperator  OutDataTypeStr=boolean  RndMeth=Simplest
  Equal1 : RelationalOperator  OutDataTypeStr=boolean  RndMeth=Simplest
  GreaterThan : RelationalOperator  OutDataTypeStr=boolean  RndMeth=Simplest
  Max : MinMax  Function=max  Inputs=3
  Mux : Mux  Inputs=3
  Mux1 : Mux  Inputs=3
  Sum : Sum  Inputs=+-
  Sum1 : Sum  Inputs=+++
  Sum2 : Sum  Inputs=|+-
  Sum3 : Sum  Inputs=|+-
  Switch : Switch  Criteria=u2 > Threshold
  VBCM_PASDRML_cm : Outport
  VBCM_PASDRMR_cm : Outport  Port=2
  KBCM_USSDis_cm : Outport  Port=3
  CheckResult : Outport  Port=4
  wires:
  GreaterThan/1 -> AND/1
  VBCM_PASDRML_cm_IN/1 -> [VBCM_PASDRML_cm_IN]
  VBCM_PASDRMR_cm_IN/1 -> [VBCM_PASDRMR_cm_IN]
  KBCM_USSDis_cm_IN/1 -> [KBCM_USSDis_cm_IN]
  AND/1 -> Switch/2, CheckResult/1
  Mux/1 -> Switch/1
  [VBCM_PASDRML_cm_IN] -> Mux/1
  [VBCM_PASDRMR_cm_IN] -> Mux/2
  [KBCM_USSDis_cm_IN] -> Mux/3
  Mux1/1 -> Switch/3
  Constant/1 -> Mux1/1
  Constant1/1 -> Mux1/2
  Switch/1 -> Demux/1
  Demux/1 -> VBCM_PASDRML_cm/1
  Demux/2 -> VBCM_PASDRMR_cm/1
  Demux/3 -> KBCM_USSDis_cm/1
  Equal/1 -> AND/2
  [VBCM_PASDRML_cm_IN] -> Max/1, Sum1/1
  [VBCM_PASDRMR_cm_IN] -> Max/2, Sum1/2
  [KBCM_USSDis_cm_IN] -> Max/3, Sum1/3
  Sum1/1 -> Sum/1
  Max/1 -> Sum/2, GreaterThan/2
  Sum/1 -> GreaterThan/1
  Constant2/1 -> Mux1/3
  Equal1/1 -> AND/3
  [VBCM_PASDRMR_cm_IN] -> Equal/1
  Constant3/1 -> Sum2/1
  Constant4/1 -> Sum2/2
  Sum2/1 -> Equal/2
  Sum3/1 -> Equal1/2
  Constant6/1 -> Sum3/2
  Constant5/1 -> Sum3/1
  [VBCM_PASDRML_cm_IN] -> Equal1/1

== system bcm/BCM/BCM/PTG/KeyDetected/Target_h ==
  VBCM_PASDRML_cm : Inport
  VBCM_PASDRMR_cm : Inport  Port=2
  KBCM_USSDis_cm : Inport  Port=3
  Data Type Conversion : DataTypeConversion
  Divide : Product  Inputs=*/
  Gain : Gain  Gain=2
  Gain1 : Gain  Gain=0.5
  Product : Product  Inputs=4
  Sqrt1 : Sqrt  SaturateOnIntegerOverflow=on
  Sum : Sum  Inputs=+-
  Sum1 : Sum  Inputs=+++
  Sum2 : Sum  Inputs=+-
  Sum3 : Sum  Inputs=+-
  Terminator : Terminator
  Target_h : Outport
  wires:
  Divide/1 -> Data Type Conversion/1, Target_h/1
  VBCM_PASDRML_cm/1 -> Sum/2, Sum1/1
  VBCM_PASDRMR_cm/1 -> Sum2/2, Sum1/2
  KBCM_USSDis_cm/1 -> Divide/2, Sum3/2, Sum1/3
  Sum1/1 -> Gain1/1
  Sum/1 -> Product/2
  Sum2/1 -> Product/3
  Sum3/1 -> Product/4
  Product/1 -> Sqrt1/1
  Sqrt1/1 -> Gain/1
  Gain/1 -> Divide/1
  Gain1/1 -> Sum3/1, Sum2/1, Sum/1, Product/1
  Data Type Conversion/1 -> Terminator/1  "VBCM_Targeth_cm"

== system bcm/BCM/BCM/PTG/KeyDetected/cosRML ==
  VBCM_PASDRML_cm : Inport
  VBCM_PASDRMR_cm : Inport  Port=2
  KBCM_USSDis_cm : Inport  Port=3
  Divide : Product  Inputs=*/
  Gain : Gain  Gain=2
  Product : Product
  Square : Math  Operator=square  SaturateOnIntegerOverflow=on
  Square1 : Math  Operator=square  SaturateOnIntegerOverflow=on
  Square2 : Math  Operator=square  SaturateOnIntegerOverflow=on
  Sum : Sum  Inputs=+-+
  cosRML : Outport
  wires:
  VBCM_PASDRML_cm/1 -> Product/1, Square/1
  VBCM_PASDRMR_cm/1 -> Square1/1
  KBCM_USSDis_cm/1 -> Product/2, Square2/1
  Square/1 -> Sum/1
  Square1/1 -> Sum/2
  Square2/1 -> Sum/3
  Product/1 -> Gain/1
  Sum/1 -> Divide/1
  Divide/1 -> cosRML/1
  Gain/1 -> Divide/2
